simulink model "model"  (R2022b)
settings: Solver=VariableStepAuto  StartTime=0.0  StopTime=10.0  RelTol=1e-3
values from neighbouring files (symbols this model uses):
  K = [kx,0 ... (first row only)    [cbf_single_obs_params.m]
  obj = [3.8,6.5]    [cbf_single_obs_params.m]
  thr = norm(v(i,:))    [cbf_centralized.m]    (also in cbf_decentralized.m; cbf_single_obs_params.m = 0.1)
  X0 = [x0;y0]    [cbf_single_obs_params.m]
  Xd = [xd;yd]    [cbf_single_obs_params.m]
  Xd_dot = [xd_dot; yd_dot]    [cbf_single_obs_params.m]
libraries: slctrlblks x1
settings Model: Creator=dorec  LastModifiedBy=dorec

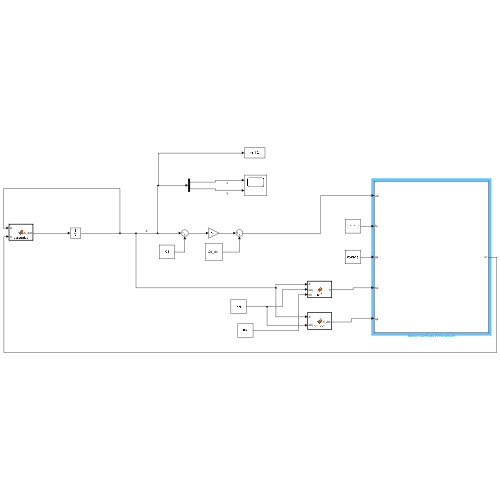
[thumbnail: Simulink's stored preview of the top-level diagram]
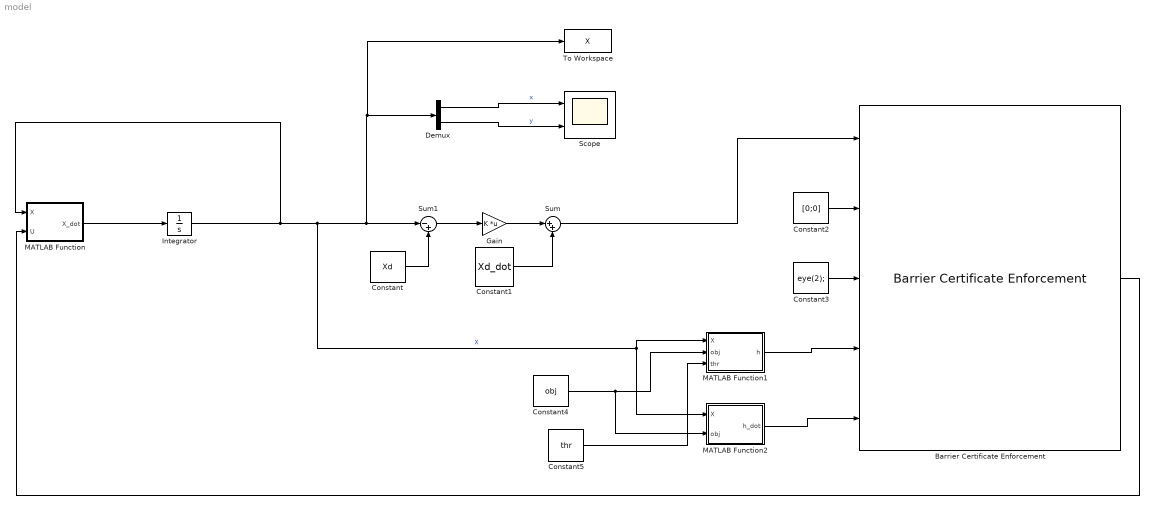
== system model ==
  Barrier Certificate Enforcement : slctrlblks/Barrier Certificate Enforcement  nx=2  nu=2  nc=1  gamma=10  beta=1  external_umax=off  external_umin=off  Ts=0.1  maxiter=200  tol=1e-6  output_exitflag=off
  Constant : Constant  Value=Xd
  Constant1 : Constant  Value=Xd_dot
  Constant2 : Constant  Value=[0;0]
  Constant3 : Constant  Value=eye(2);
  Constant4 : Constant  Value=obj
  Constant5 : Constant  Value=thr
  Demux : Demux  Outputs=2
  Gain : Gain  Gain=K  Multiplication=Matrix(K*u)
  Integrator : Integrator  InitialCondition=X0
  MATLAB Function : MATLAB Function  TreatAsAtomicUnit=on
  MATLAB Function1 : MATLAB Function  TreatAsAtomicUnit=on
  MATLAB Function2 : MATLAB Function  TreatAsAtomicUnit=on
  Scope : Scope  NumInputPorts=2
  Sum : Sum  Inputs=|++
  Sum1 : Sum  Inputs=|-+
  To Workspace : ToWorkspace  VariableName=X  SaveFormat=Timeseries  SampleTime=-1
  wires:
  Integrator/1 -> MATLAB Function2/1(X), MATLAB Function1/1(X), Sum1/1, To Workspace/1, Demux/1, MATLAB Function/1(X)  "X"
  Sum1/1 -> Gain/1
  Constant/1 -> Sum1/2
  Gain/1 -> Sum/1
  Constant1/1 -> Sum/2
  Sum/1 -> Barrier Certificate Enforcement/1
  MATLAB Function/1(X_dot) -> Integrator/1
  Demux/1 -> Scope/1  "x"
  Demux/2 -> Scope/2  "y"
  MATLAB Function1/1(h) -> Barrier Certificate Enforcement/4
  MATLAB Function2/1(h_dot) -> Barrier Certificate Enforcement/5
  Constant3/1 -> Barrier Certificate Enforcement/3
  Constant2/1 -> Barrier Certificate Enforcement/2
  Barrier Certificate Enforcement/1 -> MATLAB Function/2(U)
  Constant4/1 -> MATLAB Function1/2(obj), MATLAB Function2/2(obj)
  Constant5/1 -> MATLAB Function1/3(thr)

== matlab function model/MATLAB Function1 ==
  data: X input; obj input; thr input; h output
function h = cbf(X, obj, thr)

h = norm(X - obj) - thr;

== matlab function model/MATLAB Function ==
  data: X input; U input; X_dot output
function X_dot = dynamics(X,U)

x_dot = U(1);
y_dot = U(2);

X_dot = [x_dot; y_dot];

== matlab function model/MATLAB Function2 ==
  data: X input; h_dot output; obj input
function h_dot = cbf_dot(X, obj)

h_dot = [(X(1)-obj(1))/norm(X-obj), (X(2)-obj(2))/norm(X-obj)];
